simulink model "Lab5_LeadLag"  (R2016a)
settings: Solver=VariableStepAuto  StartTime=0.0  StopTime=30.0  RelTol=1e-3
libraries: simulink x2
settings Model: Creator=jordan  LastModifiedBy=jordan

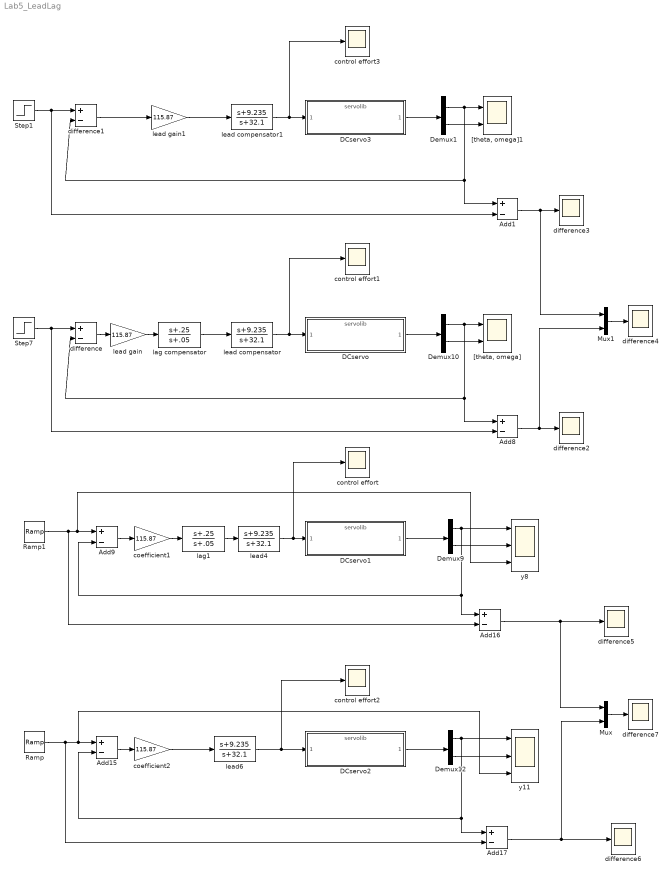
== system Lab5_LeadLag ==
  Add{1,8..9,15..17} (6 alike) : Sum  Inputs=+-
  DCservo{,1..3} (4 alike) : ModelReference  ModelNameDialog=servolib.slx  SimulationMode=Normal  ModelReferenceVersion=1.34
  Demux{1,9..10,12} (4 alike) : Demux  Outputs=2
  Mux : Mux  Inputs=2
  Mux1 : Mux  Inputs=2
  Ramp : simulink/Sources/Ramp  slope=1  start=0  X0=0
  Ramp1 : simulink/Sources/Ramp  slope=1  start=0  X0=0
  Step1 : Step  SampleTime=0
  Step7 : Step  SampleTime=0
  "[theta, omega]" : Scope  NumInputPorts=2
  "[theta, omega]1" : Scope  NumInputPorts=2
  coefficient1 : Gain  Gain=115.87
  coefficient2 : Gain  Gain=115.87
  control effort{,1..3} (4 alike) : Scope
  difference : Sum  Inputs=+-
  difference1 : Sum  Inputs=+-
  difference{2..7} (6 alike) : Scope
  lag compensator : TransferFcn  Numerator=[1 .25]  Denominator=[1 .05]
  lag1 : TransferFcn  Numerator=[1 .25]  Denominator=[1 .05]
  lead compensator : TransferFcn  Numerator=[1 9.235]  Denominator=[1 32.1]
  lead compensator1 : TransferFcn  Numerator=[1 9.235]  Denominator=[1 32.1]
  lead gain : Gain  Gain=115.87
  lead gain1 : Gain  Gain=115.87
  lead4 : TransferFcn  Numerator=[1 9.235]  Denominator=[1 32.1]
  lead6 : TransferFcn  Numerator=[1 9.235]  Denominator=[1 32.1]
  y11 : Scope  NumInputPorts=3
  y8 : Scope  NumInputPorts=3
  wires:
  lead compensator/1 -> control effort1/1, DCservo/1
  Demux10/2 -> "[theta, omega]"/2
  difference/1 -> lead gain/1
  Step7/1 -> difference/1, Add8/2
  Add8/1 -> Mux1/2, difference2/1
  Demux10/1 -> difference/2, Add8/1, "[theta, omega]"/1
  lag compensator/1 -> lead compensator/1
  lead gain/1 -> lag compensator/1
  DCservo/1 -> Demux10/1
  lead4/1 -> control effort/1, DCservo1/1
  Demux9/1 -> Add16/1, Add9/2, y8/1
  Demux9/2 -> y8/2
  Add9/1 -> coefficient1/1
  coefficient1/1 -> lag1/1
  lag1/1 -> lead4/1
  lead6/1 -> control effort2/1, DCservo2/1
  Demux12/1 -> Add15/2, Add17/1, y11/1
  Demux12/2 -> y11/2
  Add15/1 -> coefficient2/1
  coefficient2/1 -> lead6/1
  Ramp/1 -> Add17/2, y11/3, Add15/1
  Add16/1 -> Mux/1, difference5/1
  Add17/1 -> Mux/2, difference6/1
  Mux/1 -> difference7/1
  Ramp1/1 -> Add16/2, y8/3, Add9/1
  DCservo1/1 -> Demux9/1
  DCservo2/1 -> Demux12/1
  lead compensator1/1 -> control effort3/1, DCservo3/1
  Demux1/2 -> "[theta, omega]1"/2
  difference1/1 -> lead gain1/1
  Step1/1 -> difference1/1, Add1/2
  Add1/1 -> Mux1/1, difference3/1
  Demux1/1 -> difference1/2, Add1/1, "[theta, omega]1"/1
  lead gain1/1 -> lead compensator1/1
  DCservo3/1 -> Demux1/1
  Mux1/1 -> difference4/1
